simulink model "pqa_sag"  (R2024b)
settings: Solver=VariableStepAuto  StartTime=0.0  StopTime=1  RelTol=1e-3
libraries: spsVoltageMeasurementLib x2, spsACVoltageSourceLib x1, spsControlledVoltageSourceLib x1, spsCurrentMeasurementLib x1, spsGroundLib x1, spsSeriesRLCLoadLib x1, spsUniversalBridgeLib x1, sps_lib x1
settings Model: Creator=ARAVIND  LastModifiedBy=ARAVIND

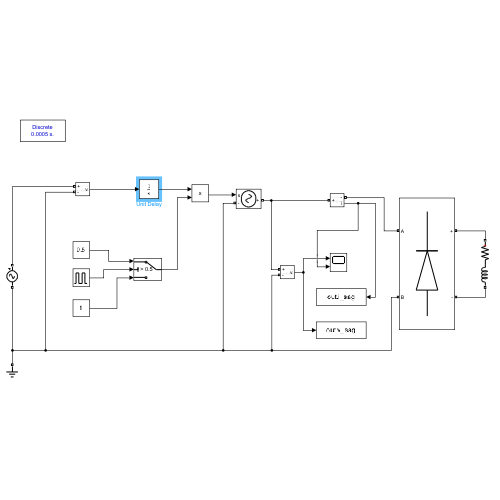
[thumbnail: Simulink's stored preview of the top-level diagram]
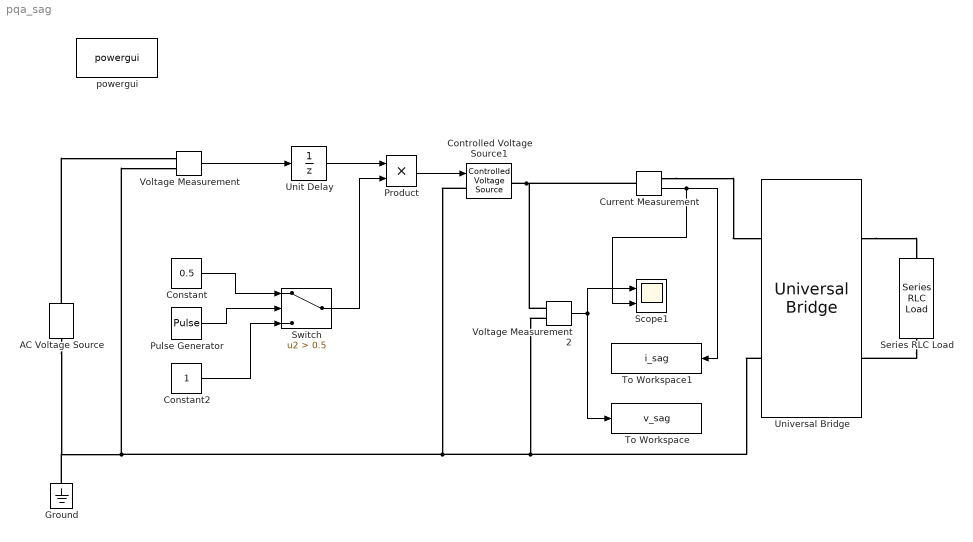
== system pqa_sag ==
  AC Voltage Source : spsACVoltageSourceLib/AC Voltage Source  Amplitude=325.27  Phase=0  Frequency=50  SampleTime=0  Measurements=None  BusType=swing  Pref=10e3  Qref=0  Qmin=-inf  Qmax=+inf
  Constant : Constant  Value=0.5
  Constant2 : Constant
  Controlled Voltage Source1 : spsControlledVoltageSourceLib/Controlled Voltage Source  Initialize=on  Source_Type=AC  Amplitude=0  Phase=0  Frequency=0  Measurements=None
  Current Measurement : spsCurrentMeasurementLib/Current Measurement  PhasorSimulation=off  OutputType=Complex  PSBequivalent=0
  Ground : spsGroundLib/Ground  LConnTagsString=a
  Product : Product
  Pulse Generator : DiscretePulseGenerator  PulseType=Time based  Period=0.4  PulseWidth=50  PhaseDelay=0.1
  Scope1 : Scope  NumInputPorts=2
  Series RLC Load : spsSeriesRLCLoadLib/Series RLC Load  LConnTagsString=a  RConnTagsString=__new0  NominalVoltage=230  NominalFrequency=50  ActivePower=1525  InductivePower=2395  CapacitivePower=0  Setx0=off  InitialVoltage=0  SetiL0=off  InitialCurrent=0  Measurements=None  LoadType=constant Z
  Switch : Switch  Criteria=u2 > Threshold  Threshold=0.5  SaturateOnIntegerOverflow=off  InputSameDT=off
  To Workspace : ToWorkspace  VariableName=v_sag  SampleTime=-1
  To Workspace1 : ToWorkspace  VariableName=i_sag  SampleTime=-1
  Unit Delay : UnitDelay  SampleTime=5e-4  HasFrameUpgradeWarning=on
  Universal Bridge : spsUniversalBridgeLib/Universal Bridge  Arms=2  SnubberResistance=1e5  SnubberCapacitance=inf  Device=Diodes  Ron=1e-3  Lon=0  ForwardVoltages="[  0  0  ]"  ForwardVoltage=0  GTOparameters=[ 10e-6 , 20e-6 ]  IGBTparameters=[ 1e-6 , 2e-6 ]  Measurements=None  Measurements_2=None  converterType=Rectifier
  Voltage Measurement : spsVoltageMeasurementLib/Voltage Measurement  PhasorSimulation=off  OutputType=Complex  PSBequivalent=0
  Voltage Measurement2 : spsVoltageMeasurementLib/Voltage Measurement  PhasorSimulation=off  OutputType=Complex  PSBequivalent=0
  powergui : sps_lib/powergui  Priority=1  SimulationMode=Discrete  SampleTime=5e-4  frequency=60  Iterations=50  frequencyindice=50  Pbase=100e6  ErrMax=1e-4  UnitsV=kV  UnitsW=MW  buscounter=0  FunctionMessages=off  echomessages=off  EnableUseOfTLC=off  CurrentSourceSwitches=off  DisableSnubberDevices=off  DisableRonSwitches=off  DisableVfSwitches=off  DisplayEquations=off  AutomaticDiscreteSolvers=off  SolverType=Tustin/Backward Euler (TBE)  Interpol=off  ExternalGateDelay=off  methode=off  Ts=100  x0status=blocks  SPID=on  SwTol=0  HookPort=off  NonlinearTolerance=1e-4  nMaxIteration=100  ContinueOnMaxIteration=off  RestoreLinks=warning  ResistiveCurrentMeasurement=off  Frange=[0:2:500]  Ylog=off  Xlog=on  ShowGrid=off  save=off  variable=ZData  structure=0  ZoomFFT=off  StartTime=0.0  cycles=1  DisplayStyle=1  fundamental=60  FreqAxis=off  MaxFrequency=1000  frequencyindicesteady=1  RmsSteady=1  display=off
  wires:
  Voltage Measurement2/1 -> Scope1/1, To Workspace/1
  Product/1 -> Controlled Voltage Source1/1
  Constant2/1 -> Switch/3
  Constant/1 -> Switch/1
  Voltage Measurement/1 -> Unit Delay/1
  Pulse Generator/1 -> Switch/2
  Unit Delay/1 -> Product/1
  Switch/1 -> Product/2
  Current Measurement/1 -> To Workspace1/1, Scope1/2
  connections:
  Universal Bridge/LConn2 -- Controlled Voltage Source1/LConn1 -- Ground/LConn1 -- AC Voltage Source/LConn1 -- Voltage Measurement/LConn2 -- Voltage Measurement2/LConn2
  Controlled Voltage Source1/RConn1 -- Voltage Measurement2/LConn1 -- Current Measurement/LConn1
  Universal Bridge/RConn1 -- Series RLC Load/LConn1
  Series RLC Load/RConn1 -- Universal Bridge/RConn2
  AC Voltage Source/RConn1 -- Voltage Measurement/LConn1
  Current Measurement/RConn1 -- Universal Bridge/LConn1
